simulink model "estimator"  (R2023b)
settings: Solver=FixedStepAuto  StartTime=0.0  StopTime=30  FixedStep=0.01  RelTol=1e-3
values from neighbouring files (symbols this model uses):
  A = [0 1 0 0 ... (first row only)    [LQR_ctp_template.m]
  B = [0; 1/M; 0; s*1/(M*L)]    [LQR_ctp_template.m]
undefined symbols (not defined in the file or in its folder): Ke
settings Model: Creator=anujsreenivasan  LastModifiedBy=anujsreenivasan

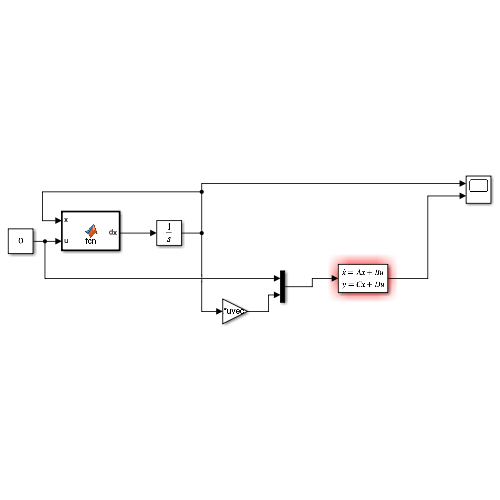
[thumbnail: Simulink's stored preview of the top-level diagram]
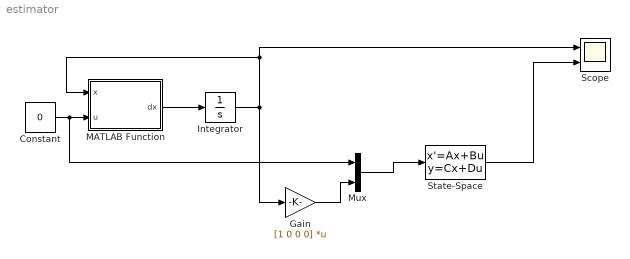
== system estimator ==
  Constant : Constant  Value=0
  Gain : Gain  Gain=[1 0 0 0]  Multiplication=Matrix(K*u) (u vector)
  Integrator : Integrator  InitialCondition=[0; 0; 0.2; 0]
  MATLAB Function : MATLAB Function  TreatAsAtomicUnit=on
  Mux : Mux  Inputs=2
  Scope : Scope  NumInputPorts=2
  State-Space : StateSpace  A=A-Ke*[1 0 0 0]  B=[B Ke]  C=eye(4)  D=0*[B Ke]  InitialCondition=[0;0;0;0]
  wires:
  MATLAB Function/1(dx) -> Integrator/1
  Integrator/1 -> Scope/1, MATLAB Function/1(x), Gain/1
  Constant/1 -> Mux/1, MATLAB Function/2(u)
  Mux/1 -> State-Space/1
  Gain/1 -> Mux/2
  State-Space/1 -> Scope/2

== matlab function estimator/MATLAB Function ==
  data: x input; u input; dx output
function dx = fcn(x,u)
dx = zeros(4,1);
m = 1; % mass of pendulum
M = 5; % mass of cart
L = 2; % length of pendulum
g = -9.81; % m/s^2
d = 10; % Ns/m
  Sx= sin(x(3));
  Cx = cos(x(3));
  D = m*L*L*(M+m*(1-Cx^2));

  dx(1,1) = x(2);
  dx(2,1) = (1/D)*(-m^2*L^2*g*Cx*Sx + m*L^2*(m*L*x(4)^2*Sx-d*x(2)))+m*L^2/D*u;
  dx(3,1) = x(4);
  dx(4,1) = (1/D)*((m+M)*m*g*L*Sx - m*L*Cx*(m*L*x(4)^2*Sx-d*x(2))) - m*L*Cx/D*u;

end
